simulink library "CRYP_MN_MASTER"  (Simulink 8.6)
settings: Solver=ode45  StartTime=0.0  StopTime=10.0  RelTol=1e-3
libraries: VIS_LIB x19, cdsEpicsOut x16, cdsFilt x12, cdsTP x12, cdsMuxMatrix x6, cdsEpicsBinIn x5, KAGRA_UTIL x1, cdsFunctionCall x1
(part 2 of 2)

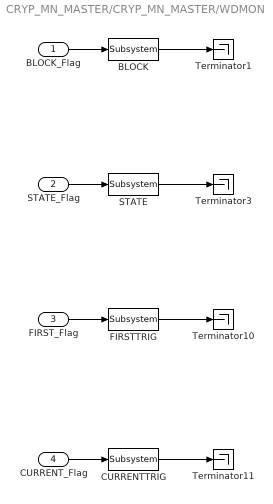
== system CRYP_MN_MASTER/CRYP_MN_MASTER/WDMON ==
  BLOCK_Flag : Inport
  STATE_Flag : Inport  Port=2
  FIRST_Flag : Inport  Port=3
  CURRENT_Flag : Inport  Port=4
  BLOCK : cdsEpicsOut/Subsystem  Tag=cdsEpicsOutput  Description="field(PREC,\"3\")"
      settings: AttributesFormatString=%<Tag>
  CURRENTTRIG : cdsEpicsOut/Subsystem  Tag=cdsEpicsOutput  Description="field(PREC,\"3\")"
      settings: AttributesFormatString=%<Tag>
  FIRSTTRIG : cdsEpicsOut/Subsystem  Tag=cdsEpicsOutput  Description="field(PREC,\"3\")"
      settings: AttributesFormatString=%<Tag>
  STATE : cdsEpicsOut/Subsystem  Tag=cdsEpicsOutput  Description="field(PREC,\"3\")"
      settings: AttributesFormatString=%<Tag>
  Terminator{1,3,10..11} (4 alike) : Terminator
  wires:
  STATE_Flag/1 -> STATE/1
  FIRST_Flag/1 -> FIRSTTRIG/1
  CURRENT_Flag/1 -> CURRENTTRIG/1
  CURRENTTRIG/1 -> Terminator11/1
  FIRSTTRIG/1 -> Terminator10/1
  BLOCK_Flag/1 -> BLOCK/1
  BLOCK/1 -> Terminator1/1
  STATE/1 -> Terminator3/1
